simulink model "IDRA_ideal"  (R2024b)
settings: Solver=VariableStepAuto  StartTime=0.0  StopTime=10.0  RelTol=1e-3
values from neighbouring files (symbols this model uses):
  Kd = eye(N_joints) * kd    [SIMULINK_pre_run.m]
  Ki = eye(N_joints) * ki    [SIMULINK_pre_run.m]
  Kp = eye(N_joints) * kp    [SIMULINK_pre_run.m]
  T_c = 1/f_c    (= 0.01)    [SIMULINK_pre_run.m]
  T_s = 1/f_s    (= 0.01)    [SIMULINK_pre_run.m]
  T_u = 1/f_u    (= 0.02)    [SIMULINK_pre_run.m]
undefined symbols (not defined in the file or in its folder): DiscIntNeverNeededParam, qd0, qdd0
settings Model: Creator=marco  LastModifiedBy=marco

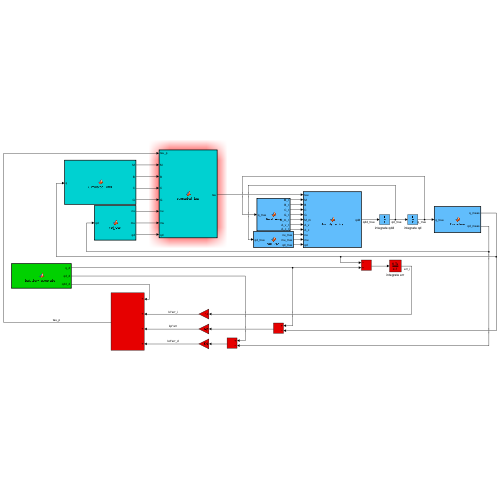
[thumbnail: Simulink's stored preview of the top-level diagram]
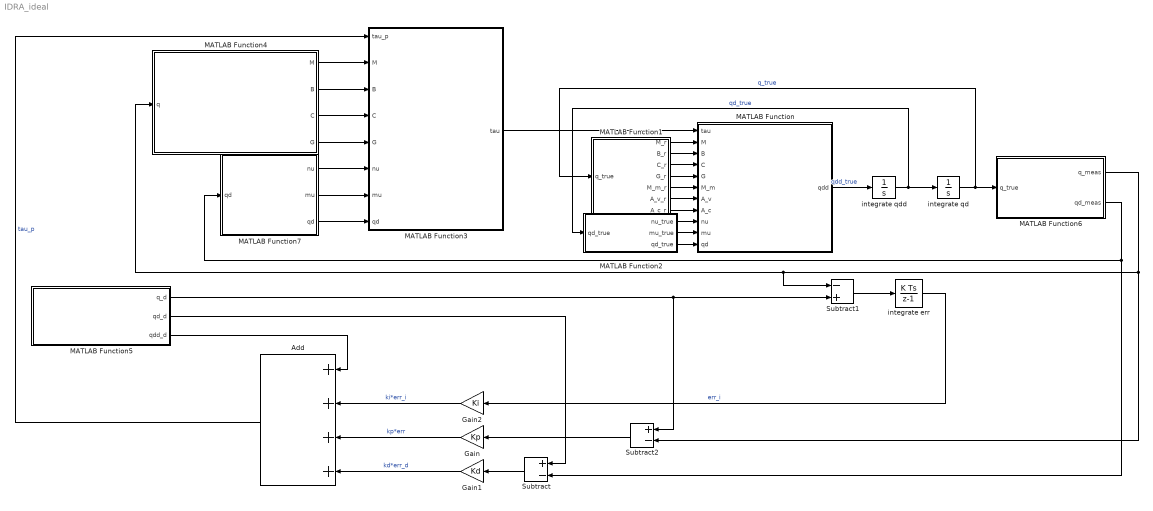
== system IDRA_ideal ==
  Add : Sum  Inputs=++++
  Gain : Gain  Gain=Kp
  Gain1 : Gain  Gain=Kd
  Gain2 : Gain  Gain=Ki
  MATLAB Function : MATLAB Function  TreatAsAtomicUnit=on
  MATLAB Function1 : MATLAB Function  TreatAsAtomicUnit=on
  MATLAB Function2 : MATLAB Function  TreatAsAtomicUnit=on
  MATLAB Function3 : MATLAB Function  TreatAsAtomicUnit=on  SystemSampleTime=T_c
  MATLAB Function4 : MATLAB Function  TreatAsAtomicUnit=on  SystemSampleTime=T_u
  MATLAB Function5 : MATLAB Function  TreatAsAtomicUnit=on
  MATLAB Function6 : MATLAB Function  TreatAsAtomicUnit=on  SystemSampleTime=T_s
  MATLAB Function7 : MATLAB Function  TreatAsAtomicUnit=on
  Subtract : Sum  Inputs=+-
  Subtract1 : Sum  Inputs=-+
  Subtract2 : Sum  Inputs=+-
  integrate err : DiscreteIntegrator  SampleTime=T_s  ICPrevOutput=DiscIntNeverNeededParam  ICPrevScaledInput=DiscIntNeverNeededParam
  integrate qd : Integrator  InitialCondition=qd0
  integrate qdd : Integrator  InitialCondition=qdd0
  wires:
  integrate err/1 -> Gain2/1  "err_i"
  MATLAB Function/1(qdd) -> integrate qdd/1  "qdd_true"
  MATLAB Function1/1(M_r) -> MATLAB Function/2(M)
  MATLAB Function1/2(B_r) -> MATLAB Function/3(B)
  MATLAB Function1/3(C_r) -> MATLAB Function/4(C)
  MATLAB Function1/4(G_r) -> MATLAB Function/5(G)
  MATLAB Function2/1(nu_true) -> MATLAB Function/9(nu)
  MATLAB Function2/2(mu_true) -> MATLAB Function/10(mu)
  MATLAB Function3/1(tau) -> MATLAB Function/1(tau)
  Add/1 -> MATLAB Function3/1(tau_p)  "tau_p"
  MATLAB Function4/3(C) -> MATLAB Function3/4(C)
  MATLAB Function4/1(M) -> MATLAB Function3/2(M)
  MATLAB Function4/2(B) -> MATLAB Function3/3(B)
  MATLAB Function4/4(G) -> MATLAB Function3/5(G)
  Subtract1/1 -> integrate err/1
  Subtract2/1 -> Gain/1
  Subtract/1 -> Gain1/1
  MATLAB Function5/1(q_d) -> Subtract2/1, Subtract1/2
  MATLAB Function5/2(qd_d) -> Subtract/1
  Gain2/1 -> Add/2  "ki*err_i"
  Gain/1 -> Add/3  "kp*err"
  Gain1/1 -> Add/4  "kd*err_d"
  MATLAB Function5/3(qdd_d) -> Add/1
  MATLAB Function2/3(qd_true) -> MATLAB Function/11(qd)
  MATLAB Function1/5(M_m_r) -> MATLAB Function/6(M_m)
  MATLAB Function1/6(A_v_r) -> MATLAB Function/7(A_v)
  MATLAB Function1/7(A_c_r) -> MATLAB Function/8(A_c)
  integrate qdd/1 -> integrate qd/1, MATLAB Function2/1("qd_true ")  "qd_true"
  integrate qd/1 -> MATLAB Function1/1(q_true), MATLAB Function6/1(q_true)  "q_true"
  MATLAB Function6/2(qd_meas) -> Subtract/2, MATLAB Function7/1("qd ")
  MATLAB Function7/1(nu) -> MATLAB Function3/6(nu)
  MATLAB Function7/2(mu) -> MATLAB Function3/7(mu)
  MATLAB Function7/3(qd) -> MATLAB Function3/8(qd)
  MATLAB Function6/1(q_meas) -> MATLAB Function4/1(q), Subtract1/1, Subtract2/2

== matlab function IDRA_ideal/MATLAB Function1 ==
  data: q_true input; M_r output; B_r output; C_r output; G_r output; M_m_r output; A_v_r output; A_c_r output
function [M_r,B_r,C_r,G_r,M_m_r,A_v_r,A_c_r] = Real_Arm(q_true)
% M B C G dipendono da modello dinamico
M_r = mass_matrix(q_true);
B_r = cor_coeff_matrix(q_true);
C_r = cent_coeff_matrix(q_true);
G_r = gravity_vector_A(q_true);
% necessita che IDRA sia stato definito nei parametri precedentemente a run
[M_m_r,A_v_r,A_c_r] = motors_effect(IDRA); % effetti presenza motore (inerzia+attrito)

end

== matlab function IDRA_ideal/MATLAB Function ==
  data: tau input; qdd output; M input; B input; C input; G input; M_m input; A_v input; A_c input; nu input; mu input; qd input
function qdd = Arm_dynamics(tau,M,B,C,G,M_m,A_v,A_c,nu,mu,qd)
% tau(dipende da modello dinamica) (M, B, C, G , M_m , A_v , A_c simulano braccio reale)
qdd = (M+M_m) \ (tau - B*nu - C*mu - G - A_v*qd - A_c.*sign(qd));
end

== matlab function IDRA_ideal/MATLAB Function2 ==
  data: nu_true output; mu_true output; qd_true input; qd_true output
function [nu_true,mu_true,qd_true] = vel_vec(qd_true)
%#codegen
nu_true = cross_joint_velocity_vector(qd_true);    % 10x1
mu_true = squared_joint_velocity_vector(qd_true);  % 5x1
end

== matlab function IDRA_ideal/MATLAB Function3 ==
  data: tau_p input; tau output; M input; B input; C input; G input; nu input; mu input; qd input
function tau = computed_tau(tau_p,M,B,C,G,nu,mu,qd)

% necessita che IDRA sia stato definito nei parametri precedentemente a run
[M_m,A_v,A_c] = motors_effect(IDRA); % effetti presenza motore (inerzia+attrito)

% ricostruzione tau
tau = (M+M_m)*tau_p + G + B*nu + C*mu + A_v*qd + A_c.*sign(qd);
end

== matlab function IDRA_ideal/MATLAB Function4 ==
  data: q input; M output; B output; C output; G output
function [M,B,C,G] = Simulated_Arm(q)
% M B C G dipendono da modello dinamico
M = mass_matrix(q);
B = cor_coeff_matrix(q);
C = cent_coeff_matrix(q);
G = gravity_vector_A(q);
end

== matlab function IDRA_ideal/MATLAB Function5 ==
  data: q_d output; qd_d output; qdd_d output
function [q_d,qd_d,qdd_d] = trajectory_generation
% ci vanno messe le matrici della traiettoria e ci va implementato sistema
% che ogni frequenza di campionamento passa a vettore relativo a tempo
% successivo
q_d = u;
qd_d = v;
qdd_d = z;
end

== matlab function IDRA_ideal/MATLAB Function6 ==
  data: q_true input; q_meas output; qd_meas output
function [q_meas, qd_meas] = Encoders(q_true)

    % Encoder assoluto: wrap -> quantize -> discrete derivative (unwrap) -> LPF
    
    % Parametri dal base workspace / model workspace:
    %   DELTA : [nx1] oppure scalar (step quantizzazione [rad])
    %   Ts    : scalar (sample time encoder/plant)
    %   tau_f : scalar (time constant LPF per qd)
    
    % ---- wrap q_true in [-pi, pi] ----
    q_true = atan2(sin(q_true), cos(q_true));
    
    % ---- quantizzazione ----
    q_meas = DELTA .* round(q_true ./ DELTA); % nella realtà ha piu senso wrappare in [0,2pi] e poi usare floor ma così è piu pulito per controllo
    
    % ---- memoria q_prev ----
    persistent q_prev y_prev is_init
    if isempty(is_init)
        q_prev  = q_meas;
        y_prev  = zeros(size(q_meas), 'like', q_meas);
        is_init = true;
    end
    
    % se cambia dimensione (es. reset o n diverso), re-init pulito
    if ~isequal(size(q_prev), size(q_meas))
        q_prev = q_meas;
        y_prev = zeros(size(q_meas), 'like', q_meas);
    end
    
    % ---- derivata discreta coerente con wrap (unwrap sulla differenza) ----
    dq = q_meas - q_prev;
    dq = atan2(sin(dq), cos(dq));     % differenza "minima" in (-pi, pi]
    qd_raw = dq ./ Ts;
    
    q_prev = q_meas;
    
    % ---- low-pass filter 1° ordine su qd ----
    if t_const <= 0
        qd_meas = qd_raw;
        y_prev  = qd_raw;
    else
        a = exp(-Ts / t_const);
        qd_meas = a .* y_prev + (1 - a) .* qd_raw;
        y_prev  = qd_meas;
    end

end

== matlab function IDRA_ideal/MATLAB Function7 ==
  data: nu output; mu output; qd input; qd output
function [nu,mu,qd] = vel_vec(qd)
%#codegen
nu = cross_joint_velocity_vector(qd);    % 10x1
mu = squared_joint_velocity_vector(qd);  % 5x1
end
